simulink model "simulink_with_signal_testing"  (R2020b)
settings: Solver=VariableStepAuto  StartTime=0.0  StopTime=inf  FixedStep=1  RelTol=1e-3
undefined symbols (not defined in the file or in its folder): sigbuilder_block
settings Model: SILPILModeSetting=veronly  EnablePacing=on  ExtModeTrigDuration=2  Creator=Ahmed Zaghloul  LastModifiedBy=Ahmed Zaghloul
settings OptimizationCC: DefaultParameterBehavior=Inlined  EnhancedBackFolding=on  PassReuseOutputArgsAs=Individual arguments  ZeroExternalMemoryAtStartup=off  ZeroInternalMemoryAtStartup=off  MaxStackSize=64  OptimizeBlockOrder=speed  DifferentSizesBufferReuse=on  OptimizationCustomize=off  EfficientTunableParamExpr=on
settings DebuggingCC: ParameterTunabilityLossMsg=error
settings HardwareCC: ProdBitPerInt=16  ProdBitPerPointer=16  ProdBitPerSizeT=16  ProdBitPerPtrDiffT=16  ProdLargestAtomicFloat=None  ProdWordSize=8  ProdHWDeviceType=Atmel->AVR
settings SFSimCC: MATLABDynamicMemAlloc=off
settings RTWCC: Description=Embedded Coder  SystemTargetFile=ert.tlc  TemplateMakefile=ert_default_tmf  Toolchain=Arduino AVR  BuildConfiguration=Faster Runs
settings CodeAppCC: ForceParamTrailComments=on  IgnoreCustomStorageClasses=off  OperatorAnnotations=on  SimulinkDataObjDesc=on  SFDataObjDesc=on  InsertBlockDesc=on
settings ERTTargetCC: SupportContinuousTime=on  ExtModeStaticAllocSize=250  InlinedParameterPlacement=NonHierarchical  ERTCustomFileTemplate=example_file_process.tlc

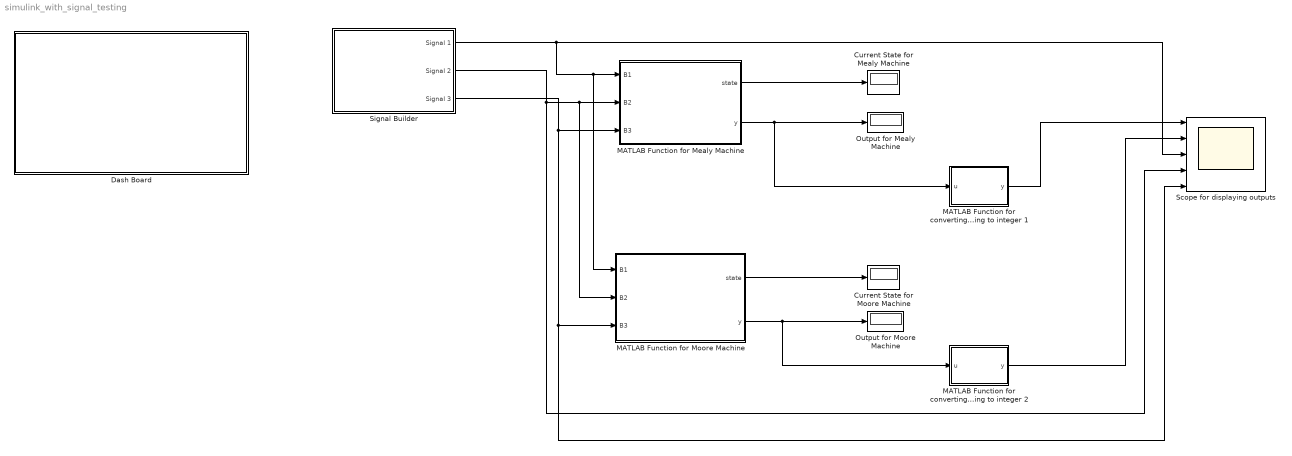
== system simulink_with_signal_testing ==
  Current State for Mealy Machine : Display
  Current State for Moore Machine : Display
  Dash Board : Subsystem
  MATLAB Function for Mealy Machine : MATLAB Function  TreatAsAtomicUnit=on
  MATLAB Function for Moore Machine : MATLAB Function  TreatAsAtomicUnit=on
  MATLAB Function for converting output string to integer 1 : MATLAB Function  TreatAsAtomicUnit=on
  MATLAB Function for converting output string to integer 2 : MATLAB Function  TreatAsAtomicUnit=on
  Output for Mealy Machine : Display
  Output for Moore Machine : Display
  Scope for displaying outputs : Scope  NumInputPorts=5
  Signal Builder : Subsystem  Tag=STV Subsys  LoadFcn=sigbuilder_block('load',[0 36 1152 555.6 ]);  StartFcn=sigbuilder_block('start');  StopFcn=sigbuilder_block('stop');  ClipboardFcn=sigbuilder_block('clipboard');  mask(Sigbuilder block){tuvar=[0:10]}
      mask help: Simulink:masks:SigbuilderBlock_MD
      mask init:
      | if ~strcmp(get_param(bdroot(gcbh),'SimulationStatus'),'stopped') tuvar = sigbuilder_block('maskInit'); end
      settings: CopyFcn=sigbuilder_block('copy');  DeleteFcn=sigbuilder_block('delete');  ModelCloseFcn=sigbuilder_block('modelClose');  PreSaveFcn=sigbuilder_block('preSave');  PauseFcn=sigbuilder_block('pause');  ContinueFcn=sigbuilder_block('continue');  NameChangeFcn=sigbuilder_block('namechange');  OpenFcn=sigbuilder_block('open',[5.4 36 1141.2 516.6 ]);  CloseFcn=sigbuilder_block('close');
      mask Display: plot(0, 0, 100, 100,[2, 2, 32, 32, 2], [68, 8, 8, 68, 68],[32, 2], [38, 38], [32, 19, 2],[53, 60, 44], [32, 17, 17, 2],[16, 16, 31, 31]);txt = getActiveGroup(gcbh);text(2, 100, txt,'verticalAlignment', 'top');
  wires:
  MATLAB Function for Moore Machine/1(state) -> Current State for Moore Machine/1
  MATLAB Function for Moore Machine/2(y) -> MATLAB Function for converting output string to integer 2/1(u), Output for Moore Machine/1
  MATLAB Function for converting output string to integer 2/1(y) -> Scope for displaying outputs/2
  MATLAB Function for Mealy Machine/1(state) -> Current State for Mealy Machine/1
  MATLAB Function for Mealy Machine/2(y) -> MATLAB Function for converting output string to integer 1/1(u), Output for Mealy Machine/1
  MATLAB Function for converting output string to integer 1/1(y) -> Scope for displaying outputs/1
  Signal Builder/2(Signal 2) -> Scope for displaying outputs/4, MATLAB Function for Moore Machine/2(B2), MATLAB Function for Mealy Machine/2(B2)
  Signal Builder/1(Signal 1) -> MATLAB Function for Moore Machine/1(B1), MATLAB Function for Mealy Machine/1(B1), Scope for displaying outputs/3
  Signal Builder/3(Signal 3) -> MATLAB Function for Moore Machine/3(B3), Scope for displaying outputs/5, MATLAB Function for Mealy Machine/3(B3)

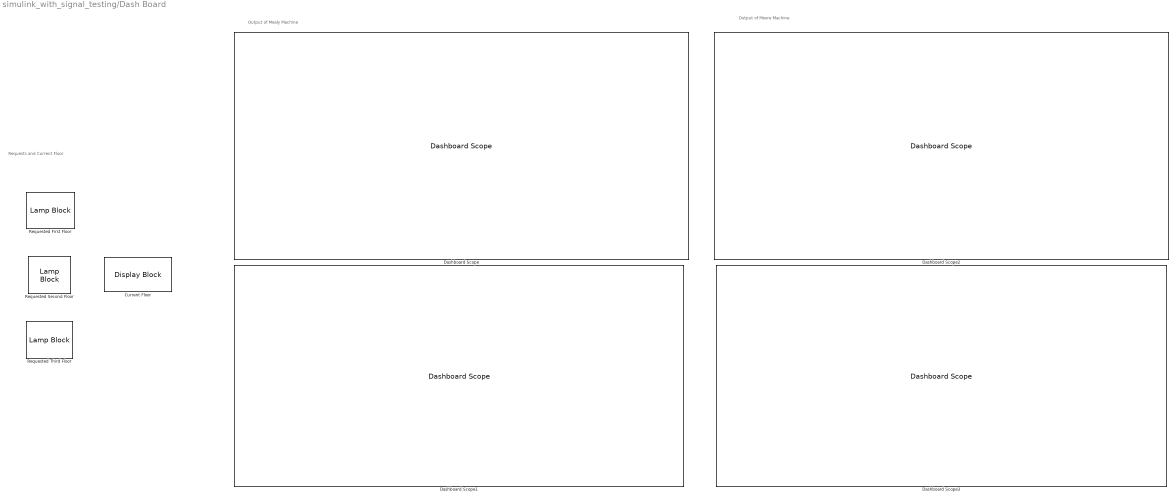
== system simulink_with_signal_testing/Dash Board ==
  note: Output of Mealy Machine
  note: Requests and Current Floor
  note: Output of Moore Machine
  Current Floor : DisplayBlock  LabelPosition=Hide  Format=short  Transparency=1
  Dashboard Scope : DashboardScope  TimeSpan=20  Ymin=-2.5  Ymax=2.5  ScaleAtStop=off
  Dashboard Scope1 : DashboardScope  TimeSpan=20  Ymin=-0.5  Ymax=1.5  ScaleAtStop=off
  Dashboard Scope2 : DashboardScope  TimeSpan=20  Ymin=-2.5  Ymax=2.5  ScaleAtStop=off
  Dashboard Scope3 : DashboardScope  TimeSpan=20  Ymin=-0.5  Ymax=1.5  ScaleAtStop=off
  Requested First Floor : LampBlock
  Requested Second Floor : LampBlock
  Requested Third Floor : LampBlock

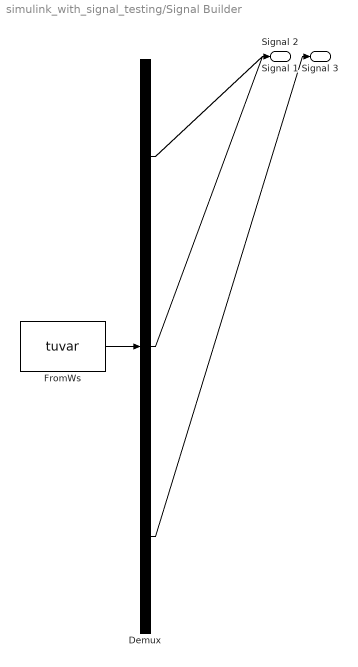
== system simulink_with_signal_testing/Signal Builder ==
  Demux : Demux  Tag=STV Demux  Outputs=3
      settings: DisplayOption=none
  FromWs : FromWorkspace  Tag=STV FromWs  VariableName=tuvar  SampleTime=0.1  OutputAfterFinalValue=Setting to zero
      SigBuilderData=|
      | common.afterFinalStr = 'Set to zero'
      | common.sampleTime = '0.1'
      | dataSet.timeRange = [0 20]
      | dataSet.name = 'Group 1'
      | sbobj.Groups.Name = 'Group 1'
      | sbobj.Groups.Signals(1).Name = 'Signal 1'
      | sbobj.Groups.Signals(1).XData = [0 1 1 3 3 6 8 10 10 12 12 14 16 18 20]
      | sbobj.Groups.Signals(1).YData = [0 0 1 1 0 0 0 0 1 1 0 0 0 0 0]
      | sbobj.Groups.Signals(2).Name = 'Signal 2'
      | sbobj.Groups.Signals(2).XData = [0 4 4 6 6 20]
      | sbobj.Groups.Signals(2).YData = [0 0 1 1 0 0]
      | sbobj.Groups.Signals(3).Name = 'Signal 3'
      | sbobj.Groups.Signals(3).XData = [0 2 4 6 7 7 9 9 12 13 13 15 15 18 20]
      | sbobj.Groups.Signals(3).YData = [0 0 0 0 0 1 1 0 0 0 1 1 0 0 0]
      | sbobj.Groups.TimeRange = [0 20]
  Signal 1 : Outport  Tag=STV Outport
  Signal 2 : Outport  Tag=STV Outport  Port=2
  Signal 3 : Outport  Tag=STV Outport  Port=3
  wires:
  FromWs/1 -> Demux/1
  Demux/1 -> Signal 1/1
  Demux/2 -> Signal 2/1
  Demux/3 -> Signal 3/1

== matlab function simulink_with_signal_testing/MATLAB Function for Moore Machine ==
  data: state output; B1 input; y output; B2 input; B3 input
function [state ,y] = fcn(B1,B2,B3)
persistent current_state
if(isempty(current_state))
    current_state = 1;
end
switch current_state
    case 1
        if(B1)
            current_state = 1;
        elseif(B2)
            current_state = 4;
        elseif(B3)
            current_state = 6;
        end
    case 2
        if(B1)
            current_state = 5;
        elseif(B2)
            current_state = 2;
        elseif(B3)
            current_state = 8;
        end
    case 3
        if(B1)
            current_state = 7;
        elseif(B2)
            current_state = 9;
        elseif(B3)
            current_state = 3;
        end
    case 4
        if(B2)
            current_state = 2;
        end
    case 5
        if(B1)
            current_state = 1;
        end
    case 6
        if(B3)
            current_state = 3;
        end  
    case 7
        if(B1)
            current_state = 1;
        end  
    case 8
        if(B3)
            current_state = 3;
        end  
    case 9
        if(B2)
            current_state = 2;
        end  
end
switch current_state
    case 1
        y = "s";
    case 2
        y = "s";
    case 3
        y = "s";
    case 4
        y = "u1";
    case 5
        y = "u1";
    case 6
        y = "u2";
    case 7
        y = "d2";
    case 8
        y = "u1";
    otherwise
        y = "d1";
end
state = current_state;
end

== matlab function simulink_with_signal_testing/MATLAB Function for Mealy Machine ==
  data: state output; B1 input; y output; B2 input; B3 input
function [state,y] = fcn(B1,B2,B3)
persistent current_state
if(isempty(current_state))
    current_state = 1;
end
switch current_state
    case 1
        if(B2)
            current_state = 2;
            y = "u1";
        elseif(B3)
            current_state = 3;
            y = "u2";
        else
            current_state = 1;
            y = "s";
        end
    case 2
        if(B1)
            current_state = 1;
            y = "d1";
        elseif(B3)
            current_state = 3;
            y = "u1";
        else
            current_state = 2;
            y = "s";
        end
    otherwise
        if(B1)
            current_state = 1;
            y = "d2";
        elseif(B2)
            current_state = 2;
            y = "d1";
        else
            current_state = 3;
            y = "s";
        end
end
state = current_state;
end

== matlab function simulink_with_signal_testing/MATLAB Function for converting output string to integer 1 ==
  data: u input; y output
function y = fcn(u)
if u == "s"
    y = 0;
elseif u == "u1"
    y = 1;
elseif u == "u2"
    y = 2;
elseif u == "d1"
    y = -1;
else
    y = -2;
end

== matlab function simulink_with_signal_testing/MATLAB Function for converting output string to integer 2 ==
  data: u input; y output
function y = fcn(u)
if u == "s"
    y = 0;
elseif u == "u1"
    y = 1;
elseif u == "u2"
    y = 2;
elseif u == "d1"
    y = -1;
else
    y = -2;
end
